simulink model "closeLoop"  (R2024a)
settings: Solver=ode45  StartTime=0.0  StopTime=1000  FixedStep=1E-4  RelTol=1e-3
values from neighbouring files (symbols this model uses):
  gamma_p = 0.1    [simulationParameters.m]    (also in untitled10.m)
  Kp_init = 1    [simulationParameters.m]    (also in untitled10.m)
undefined symbols (not defined in the file or in its folder): adap, init, motor
libraries: slpidlib x1
settings Model: Creator=b_ant  LastModifiedBy=b_ant
settings DataIOCC: SaveFormat=Array

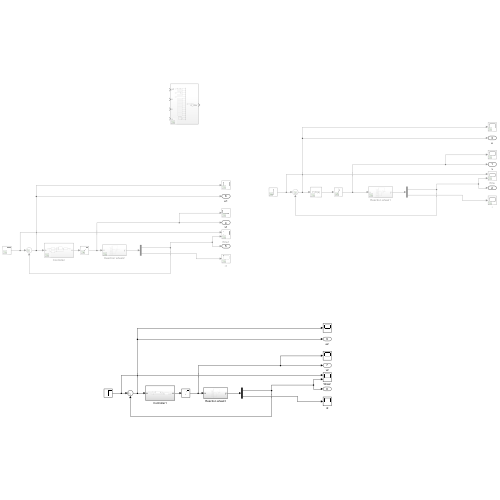
[thumbnail: Simulink's stored preview of the top-level diagram]
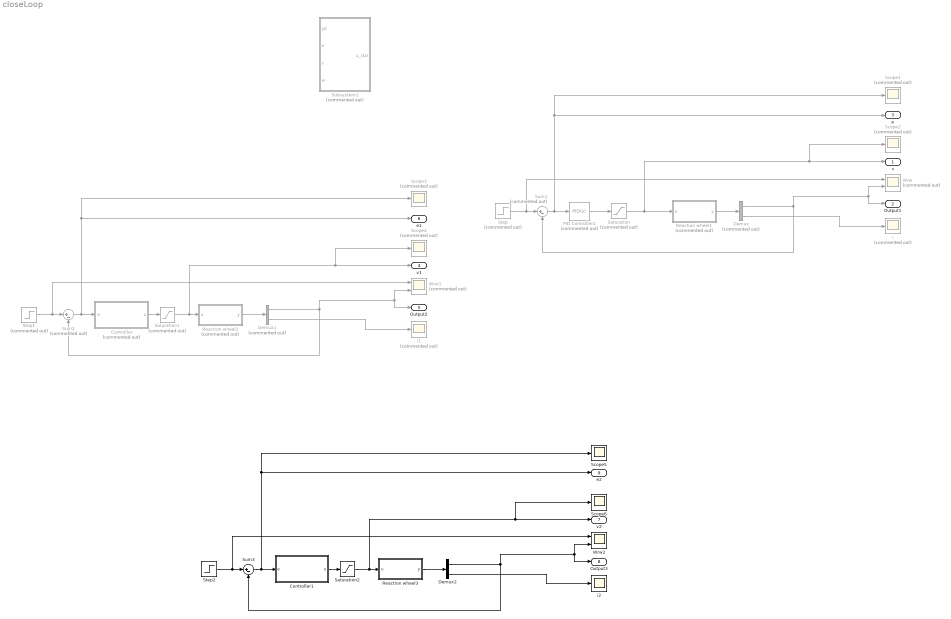
== system closeLoop ==
  Controller : Subsystem  Commented=on
  Controller1 : Subsystem
  Demux : Demux  Commented=on  Outputs=2
  Demux1 : Demux  Commented=on  Outputs=2
  Demux2 : Demux  Outputs=2
  PID Controller1 : slpidlib/PID Controller  Commented=on  Controller=PID  Form=Parallel  TimeDomain=Continuous-time  UseExternalTs=off  SampleTime=-1  IntegratorMethod=Forward Euler  FilterMethod=Forward Euler  ControllerParametersSource=internal  P=0.0125748602658066  I=0.0107348710799452  UseKiTs=off  D=0  UseExternalDerivativeSource=off  N=100  UseFilter=on  TunerSelectOption=Transfer Function Based (PID Tuner App)  InitialConditionSource=internal  InitialConditionForIntegrator=0  InitialConditionForFilter=0  DifferentiatorICPrevScaledInput=0  ExternalReset=none  TrackingMode=off  Kt=1  LimitOutput=off  SatLimitsSource=internal  UpperSaturationLimit=inf  LowerSaturationLimit=-inf  LinearizeAsGain=on  AntiWindupMode=none  Kb=1  LimitIntegrator=off  UpperIntegratorSaturationLimit=inf  LowerIntegratorSaturationLimit=-inf  POutMin=[]  POutMax=[]  IOutMin=[]  IOutMax=[]  DOutMin=[]  DOutMax=[]  NOutMin=[]  NOutMax=[]  SumOutMin=[]  SumOutMax=[]  SaturationOutMin=[]  SaturationOutMax=[]  PParamMin=[]  PParamMax=[]  IParamMin=[]  IParamMax=[]  DParamMin=[]  DParamMax=[]  NParamMin=[]  NParamMax=[]  KbParamMin=[]  KbParamMax=[]  KtParamMin=[]  KtParamMax=[]  KbOutMin=[]  KbOutMax=[]  KtOutMin=[]  KtOutMax=[]  IntegratorOutMin=[]  IntegratorOutMax=[]  FilterOutMin=[]  FilterOutMax=[]  SumI1OutMin=[]  SumI1OutMax=[]  SumI2OutMin=[]  SumI2OutMax=[]  SumI3OutMin=[]  SumI3OutMax=[]  SumI4OutMin=[]  SumI4OutMax=[]  SumDOutMin=[]  SumDOutMax=[]  DifferentiatorOutMin=[]  DifferentiatorOutMax=[]  FilterDiffOutCoefMin=[]  FilterDiffOutCoefMax=[]  ReciprocalOutMin=[]  ReciprocalOutMax=[]  SumDenOutMin=[]  SumDenOutMax=[]  SumNumOutMin=[]  SumNumOutMax=[]  DivideOutMin=[]  DivideOutMax=[]  UdiffTsProdOutMin=[]  UdiffTsProdOutMax=[]  NTsProdOutMin=[]  NTsProdOutMax=[]  UintegralTsProdOutMin=[]  UintegralTsProdOutMax=[]  UngainTsProdOutMin=[]  UngainTsProdOutMax=[]  ClampingZeroOutDataTypeStr=Inherit: Inherit via back propagation  ClampingZeroOutMin=[]  ClampingZeroOutMax=[]  FilterDenConstantOutDataTypeStr=Inherit: Inherit via back propagation  FilterDenConstantOutMin=[]  FilterDenConstantOutMax=[]  PCopyOutDataTypeStr=Inherit: Inherit via back propagation  PCopyOutMin=[]  PCopyOutMax=[]  NCopyOutDataTypeStr=Inherit: Inherit via back propagation  NCopyOutMin=[]  NCopyOutMax=[]  IntegratorContinuousStateAttributes=''  IntegratorStateMustResolveToSignalObject=off  IntegratorRTWStateStorageClass=Auto  FilterContinuousStateAttributes=''  FilterStateMustResolveToSignalObject=off  FilterRTWStateStorageClass=Auto  ParallelPVariant=InternalParameters  IdealPVariant=Disabled  IVariant=InternalParameters  DVariant=InternalParameters  IntegratorVariant=Continuous  SatVariant=Disabled  AWVariant=Passthrough  PCopyVariant=Disabled  TRVariant=Disabled  FdbkBlocksVariant=Forward  IdealPFdbkVariant=Disabled  SatFdbkVariant=Disabled  DerivativeFilterVariant=ContFilter  NVariant=InternalParameters  NCopyVariant=Disabled  FilterICVariant=InternalICsFilter  IntegratorICVariant=InternalICs  ExternalResetVariant=Disabled  TRSumVariant=Passthrough  SumFdbkVariant=Disabled  SumVariant=Sum_PID  TsampFilterVariant=InternalTs  TsampNgainVariant=Passthrough  TsampIntegralVariant=Disabled_SignalSpec  ExternalSaturationOutDataTypeStr=Inherit: Same as second input  DerivativeSourceVariant=ErrorSignal
  Reaction wheel1 : Subsystem  Commented=on
  Reaction wheel2 : Subsystem  Commented=on
  Reaction wheel3 : Subsystem
  Saturation : Saturate  Commented=on  UpperLimit=12  LowerLimit=-12
  Saturation1 : Saturate  Commented=on  UpperLimit=12  LowerLimit=-12
  Saturation2 : Saturate  UpperLimit=12  LowerLimit=-12
  Scope{1..4} (4 alike) : Scope  Commented=on
  Scope5 : Scope
  Scope6 : Scope
  Step : Step  Commented=on  After=100  SampleTime=0
  Step1 : Step  Commented=on  After=100  SampleTime=0
  Step2 : Step  After=100  SampleTime=0
  Subsystem1 : Subsystem  Commented=on
  Sum1 : Sum  Commented=on  Inputs=|+-
  Sum2 : Sum  Commented=on  Inputs=|+-
  Sum3 : Sum  Inputs=|+-
  Wrw : Scope  Commented=on  NumInputPorts=2
  Wrw1 : Scope  Commented=on  NumInputPorts=2
  Wrw2 : Scope  NumInputPorts=2
  i : Scope  Commented=on
  i1 : Scope  Commented=on
  i2 : Scope
  v : Outport
  Output1 : Outport  Port=2
  e : Outport  Port=3
  v1 : Outport  Port=4
  Output2 : Outport  Port=5
  e1 : Outport  Port=6
  v2 : Outport  Port=7
  Output3 : Outport  Port=8
  e2 : Outport  Port=9
  wires:
  Demux/1 -> Output1/1, Wrw/2, Sum1/2
  Demux/2 -> i/1
  Reaction wheel1/1(y) -> Demux/1
  Step/1 -> Wrw/1, Sum1/1
  Sum1/1 -> PID Controller1/1, e/1, Scope1/1
  PID Controller1/1 -> Saturation/1
  Saturation/1 -> Scope2/1, v/1, Reaction wheel1/1(u)
  Saturation1/1 -> Scope4/1, v1/1, Reaction wheel2/1(u)
  Step1/1 -> Wrw1/1, Sum2/1
  Reaction wheel2/1(y) -> Demux1/1
  Sum2/1 -> Controller/1(e), e1/1, Scope3/1
  Controller/1(u) -> Saturation1/1
  Demux1/1 -> Output2/1, Wrw1/2, Sum2/2
  Demux1/2 -> i1/1
  Sum3/1 -> Controller1/1(e), e2/1, Scope5/1
  Reaction wheel3/1(y) -> Demux2/1
  Demux2/1 -> Output3/1, Wrw2/2, Sum3/2
  Controller1/1(u) -> Saturation2/1
  Demux2/2 -> i2/1
  Step2/1 -> Wrw2/1, Sum3/1
  Saturation2/1 -> Scope6/1, v2/1, Reaction wheel3/1(u)

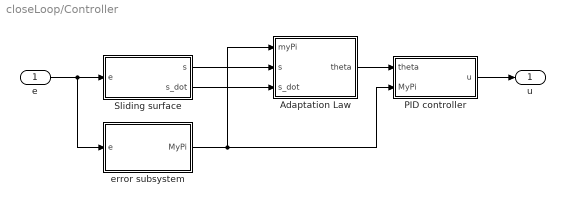
== system closeLoop/Controller ==
  e : Inport
  Adaptation Law : Subsystem  mask{alpha=adap.alpha, beta=adap.beta, epsilon=adap.epsilon, n=adap.n, kd0=adap.kd_init, ki0=adap.ki_init, kp0=adap.kp_init}
      mask prompts: kd0 "kd_0:"; ki0 "ki_0:"; kp0 "kp_0:"
      mask TypeOptions alpha: alpha/Value
      mask TypeOptions beta: beta/Value
      mask TypeOptions epsilon: epsilon/Value
      mask TypeOptions n: n/Value
      mask TypeOptions kd0: kd0/Value
      mask TypeOptions ki0: ki0/Value
      mask TypeOptions kp0: kp0/Value
  PID controller : Subsystem
  Sliding surface : Subsystem  mask{Gain=adap.lambda}
      mask prompts: Gain "Simulink:blkprm_prompts:GainGain"
      mask TypeOptions Gain: Gain/Gain
      mask DialogControl Gain Prompt: Gain:
  error subsystem : Subsystem
  u : Outport
  wires:
  Sliding surface/1(s) -> Adaptation Law/2(s)
  Sliding surface/2(s_dot) -> Adaptation Law/3(s_dot)
  PID controller/1(u) -> u/1
  Adaptation Law/1(theta) -> PID controller/1(theta)
  error subsystem/1(MyPi) -> PID controller/2(MyPi), Adaptation Law/1(myPi)
  e/1 -> error subsystem/1(e), Sliding surface/1(e)

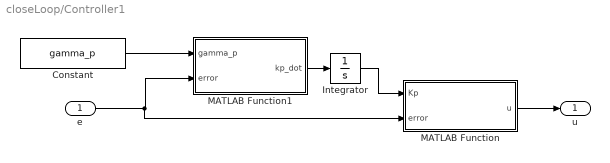
== system closeLoop/Controller1 ==
  e : Inport
  Constant : Constant  Value=gamma_p
  Integrator : Integrator  InitialCondition=Kp_init
  MATLAB Function : MATLAB Function  TreatAsAtomicUnit=on
  MATLAB Function1 : MATLAB Function  TreatAsAtomicUnit=on
  u : Outport
  wires:
  MATLAB Function/1(u) -> u/1
  MATLAB Function1/1(kp_dot) -> Integrator/1
  Integrator/1 -> MATLAB Function/1(Kp)
  e/1 -> MATLAB Function/2(error), MATLAB Function1/2(error)
  Constant/1 -> MATLAB Function1/1(gamma_p)

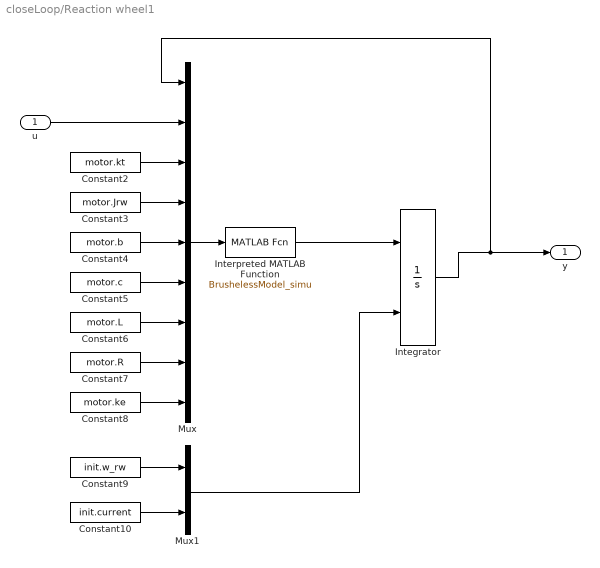
== system closeLoop/Reaction wheel1 ==
  u : Inport
  Constant10 : Constant  Value=init.current
  Constant2 : Constant  Value=motor.kt
  Constant3 : Constant  Value=motor.Jrw
  Constant4 : Constant  Value=motor.b
  Constant5 : Constant  Value=motor.c
  Constant6 : Constant  Value=motor.L
  Constant7 : Constant  Value=motor.R
  Constant8 : Constant  Value=motor.ke
  Constant9 : Constant  Value=init.w_rw
  Integrator : Integrator  InitialConditionSource=external
  Interpreted MATLAB Function : MATLABFcn  MATLABFcn=BrushelessModel_simu  OutputDimensions=2
  Mux : Mux  Inputs=9
  Mux1 : Mux  Inputs=2
  y : Outport
  wires:
  Interpreted MATLAB Function/1 -> Integrator/1
  Constant8/1 -> Mux/9
  Integrator/1 -> Mux/1, y/1
  Constant10/1 -> Mux1/2
  Constant9/1 -> Mux1/1
  Mux/1 -> Interpreted MATLAB Function/1
  Mux1/1 -> Integrator/2
  u/1 -> Mux/2
  Constant2/1 -> Mux/3
  Constant3/1 -> Mux/4
  Constant4/1 -> Mux/5
  Constant5/1 -> Mux/6
  Constant6/1 -> Mux/7
  Constant7/1 -> Mux/8

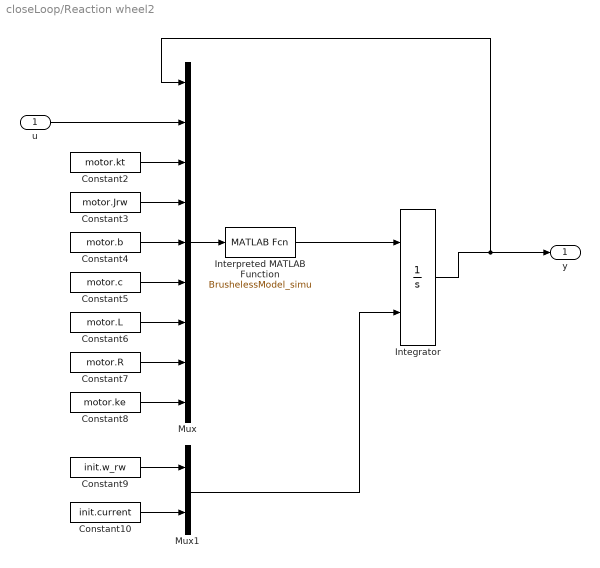
== system closeLoop/Reaction wheel2 ==
  u : Inport
  Constant10 : Constant  Value=init.current
  Constant2 : Constant  Value=motor.kt
  Constant3 : Constant  Value=motor.Jrw
  Constant4 : Constant  Value=motor.b
  Constant5 : Constant  Value=motor.c
  Constant6 : Constant  Value=motor.L
  Constant7 : Constant  Value=motor.R
  Constant8 : Constant  Value=motor.ke
  Constant9 : Constant  Value=init.w_rw
  Integrator : Integrator  InitialConditionSource=external
  Interpreted MATLAB Function : MATLABFcn  MATLABFcn=BrushelessModel_simu  OutputDimensions=2
  Mux : Mux  Inputs=9
  Mux1 : Mux  Inputs=2
  y : Outport
  wires:
  Interpreted MATLAB Function/1 -> Integrator/1
  Constant8/1 -> Mux/9
  Integrator/1 -> Mux/1, y/1
  Constant10/1 -> Mux1/2
  Constant9/1 -> Mux1/1
  Mux/1 -> Interpreted MATLAB Function/1
  Mux1/1 -> Integrator/2
  u/1 -> Mux/2
  Constant2/1 -> Mux/3
  Constant3/1 -> Mux/4
  Constant4/1 -> Mux/5
  Constant5/1 -> Mux/6
  Constant6/1 -> Mux/7
  Constant7/1 -> Mux/8

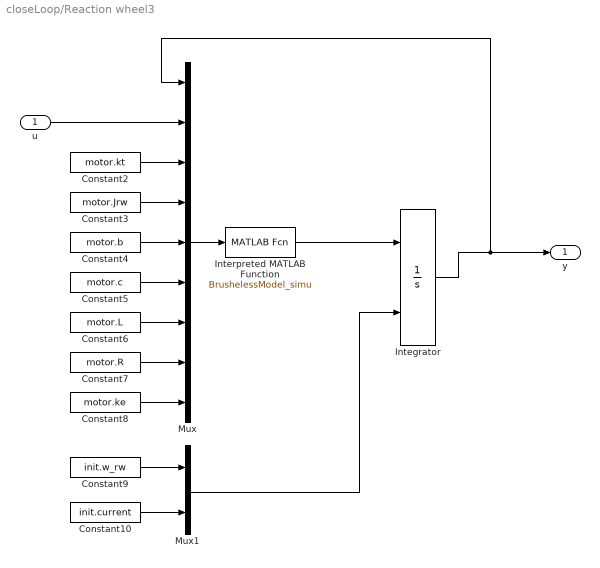
== system closeLoop/Reaction wheel3 ==
  u : Inport
  Constant10 : Constant  Value=init.current
  Constant2 : Constant  Value=motor.kt
  Constant3 : Constant  Value=motor.Jrw
  Constant4 : Constant  Value=motor.b
  Constant5 : Constant  Value=motor.c
  Constant6 : Constant  Value=motor.L
  Constant7 : Constant  Value=motor.R
  Constant8 : Constant  Value=motor.ke
  Constant9 : Constant  Value=init.w_rw
  Integrator : Integrator  InitialConditionSource=external
  Interpreted MATLAB Function : MATLABFcn  MATLABFcn=BrushelessModel_simu  OutputDimensions=2
  Mux : Mux  Inputs=9
  Mux1 : Mux  Inputs=2
  y : Outport
  wires:
  Interpreted MATLAB Function/1 -> Integrator/1
  Constant8/1 -> Mux/9
  Integrator/1 -> Mux/1, y/1
  Constant10/1 -> Mux1/2
  Constant9/1 -> Mux1/1
  Mux/1 -> Interpreted MATLAB Function/1
  Mux1/1 -> Integrator/2
  u/1 -> Mux/2
  Constant2/1 -> Mux/3
  Constant3/1 -> Mux/4
  Constant4/1 -> Mux/5
  Constant5/1 -> Mux/6
  Constant6/1 -> Mux/7
  Constant7/1 -> Mux/8

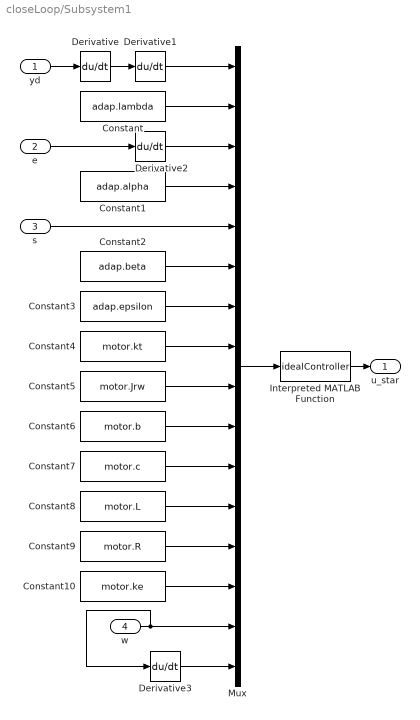
== system closeLoop/Subsystem1 ==
  yd : Inport
  e : Inport  Port=2
  s : Inport  Port=3
  w : Inport  Port=4
  Constant : Constant  Value=adap.lambda
  Constant1 : Constant  Value=adap.alpha
  Constant10 : Constant  Value=motor.ke
  Constant2 : Constant  Value=adap.beta
  Constant3 : Constant  Value=adap.epsilon
  Constant4 : Constant  Value=motor.kt
  Constant5 : Constant  Value=motor.Jrw
  Constant6 : Constant  Value=motor.b
  Constant7 : Constant  Value=motor.c
  Constant8 : Constant  Value=motor.L
  Constant9 : Constant  Value=motor.R
  Derivative{,1..3} (4 alike) : Derivative
  Interpreted MATLAB Function : MATLABFcn  MATLABFcn=idealController
  Mux : Mux  Inputs=16
  u_star : Outport
  wires:
  Constant10/1 -> Mux/14
  Interpreted MATLAB Function/1 -> u_star/1
  Derivative3/1 -> Mux/16
  Constant9/1 -> Mux/13
  Constant7/1 -> Mux/11
  Constant6/1 -> Mux/10
  Constant8/1 -> Mux/12
  Constant4/1 -> Mux/8
  Constant2/1 -> Mux/6
  s/1 -> Mux/5
  e/1 -> Derivative2/1
  Derivative/1 -> Derivative1/1
  Constant5/1 -> Mux/9
  Constant3/1 -> Mux/7
  Constant/1 -> Mux/2
  Derivative2/1 -> Mux/3
  yd/1 -> Derivative/1
  Constant1/1 -> Mux/4
  w/1 -> Mux/15, Derivative3/1
  Mux/1 -> Interpreted MATLAB Function/1
  Derivative1/1 -> Mux/1

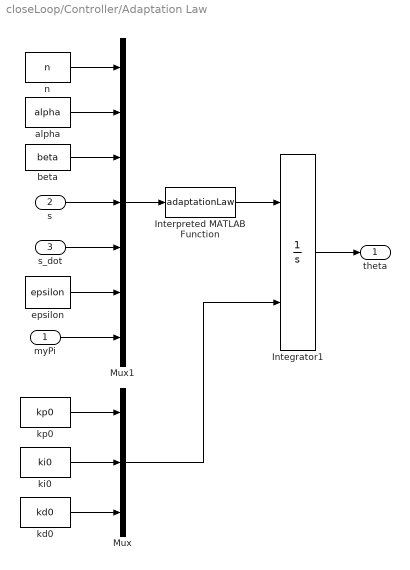
== system closeLoop/Controller/Adaptation Law ==
  myPi : Inport
  s : Inport  Port=2
  s_dot : Inport  Port=3
  Integrator1 : Integrator  InitialConditionSource=external  InitialCondition=[1.460477259865257e-04,6.548069875818259e-05,0]
  Interpreted MATLAB Function : MATLABFcn  MATLABFcn=adaptationLaw
  Mux : Mux  Inputs=3
  Mux1 : Mux  Inputs=7
  alpha : Constant  Value=alpha
  beta : Constant  Value=beta
  epsilon : Constant  Value=epsilon
  kd0 : Constant  Value=kd0
  ki0 : Constant  Value=ki0
  kp0 : Constant  Value=kp0
  n : Constant  Value=n
  theta : Outport
  wires:
  alpha/1 -> Mux1/2
  Interpreted MATLAB Function/1 -> Integrator1/1
  myPi/1 -> Mux1/7
  s/1 -> Mux1/4
  epsilon/1 -> Mux1/6
  Integrator1/1 -> theta/1
  s_dot/1 -> Mux1/5
  beta/1 -> Mux1/3
  Mux1/1 -> Interpreted MATLAB Function/1
  n/1 -> Mux1/1
  ki0/1 -> Mux/2
  Mux/1 -> Integrator1/2
  kp0/1 -> Mux/1
  kd0/1 -> Mux/3

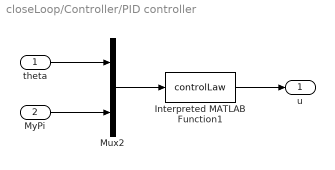
== system closeLoop/Controller/PID controller ==
  theta : Inport
  MyPi : Inport  Port=2
  Interpreted MATLAB Function1 : MATLABFcn  MATLABFcn=controlLaw  OutputDimensions=1
  Mux2 : Mux  Inputs=2
  u : Outport
  wires:
  Mux2/1 -> Interpreted MATLAB Function1/1
  theta/1 -> Mux2/1
  Interpreted MATLAB Function1/1 -> u/1
  MyPi/1 -> Mux2/2

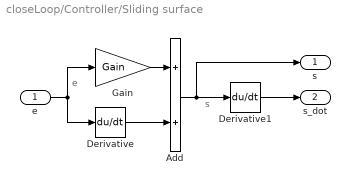
== system closeLoop/Controller/Sliding surface ==
  note: s
  note: e
  e : Inport
  Add : Sum
  Derivative : Derivative
  Derivative1 : Derivative
  Gain : Gain  Gain=Gain
  s : Outport
  s_dot : Outport  Port=2
  wires:
  Add/1 -> s/1, Derivative1/1
  Gain/1 -> Add/1
  e/1 -> Derivative/1, Gain/1
  Derivative/1 -> Add/2
  Derivative1/1 -> s_dot/1

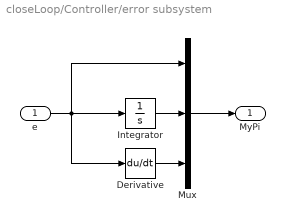
== system closeLoop/Controller/error subsystem ==
  e : Inport
  Derivative : Derivative
  Integrator : Integrator
  Mux : Mux  Inputs=3
  MyPi : Outport
  wires:
  e/1 -> Derivative/1, Mux/1, Integrator/1
  Integrator/1 -> Mux/2
  Mux/1 -> MyPi/1
  Derivative/1 -> Mux/3

== matlab function closeLoop/Controller1/MATLAB Function ==
  data: Kp input; u output; error input
function u = P_control(Kp,error)
    u = Kp * error;
end

== matlab function closeLoop/Controller1/MATLAB Function1 ==
  data: gamma_p input; kp_dot output; error input
function kp_dot = fcn(gamma_p,error)
    kp_dot = gamma_p * abs(error);
end
